simulink model "Third_Simulation"  (R2020a)
settings: Solver=VariableStepAuto  StartTime=0.0  StopTime=1  RelTol=1e-3
undefined symbols (not defined in the file): D1, Delta
libraries: powerlib x7
settings Model: Creator=amnja  LastModifiedBy=amnja

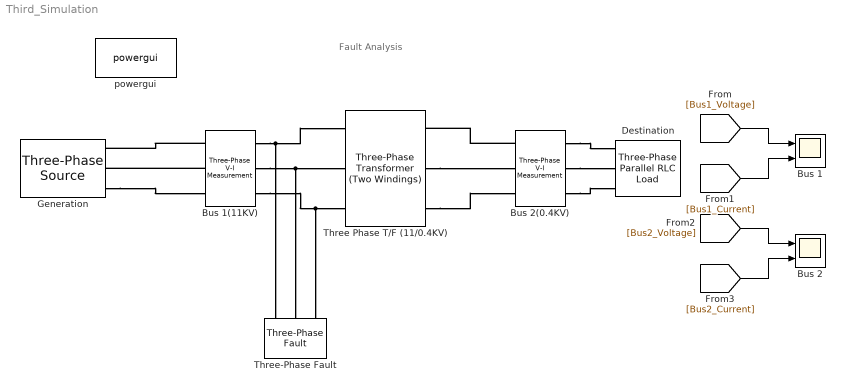
== system Third_Simulation ==
  note: Fault Analysis
  Bus 1 : Scope  NumInputPorts=2
  Bus 1(11KV) : powerlib/Measurements/Three-Phase V-I Measurement  VoltageMeasurement=phase-to-ground  SetLabelV=on  LabelV=Bus1_Voltage  Vpu=off  VpuLL=off  CurrentMeasurement=yes  SetLabelI=on  LabelI=Bus1_Current  Ipu=off  Pbase=100e6  Vbase=500e3  OutputType=Complex  PhasorSimulation=off  PSBequivalent=0
  Bus 2 : Scope  NumInputPorts=2
  Bus 2(0.4KV) : powerlib/Measurements/Three-Phase V-I Measurement  VoltageMeasurement=phase-to-ground  SetLabelV=on  LabelV=Bus2_Voltage  Vpu=off  VpuLL=off  CurrentMeasurement=yes  SetLabelI=on  LabelI=Bus2_Current  Ipu=off  Pbase=100e6  Vbase=500e3  OutputType=Complex  PhasorSimulation=off  PSBequivalent=0
  Destination : powerlib/Elements/Three-Phase Parallel RLC Load  LConnTagsString=A|B|C  Configuration=Y (grounded)  NominalVoltage=0.4e3  Vabc=[1e3 1e3 1e3]  Vabcp=[1e3 1e3 1e3]  NominalFrequency=50  UnbalancedPower=off  ActivePower=10e3  InductivePower=100  CapacitivePower=0  Pabc=[10e3 9e3 11e3]  QLabc=[100 90 110]  QCabc=[100 90 110]  Pabcp=[10e3 9e3 11e3]  QLabcp=[100 90 110]  QCabcp=[100 90 110]  Measurements=None  LoadType=constant Z
  Generation : powerlib/Electrical Sources/Three-Phase Source  InternalConnection=Yg  VoltagePhases=off  Voltage=11e3  PhaseAngle=0  Voltage_phases=[25e3 25e3 25e3]/sqrt(3)  PhaseAngles_phases=[0 -120 +120]  Frequency=50  NonIdealSource=on  SpecifyImpedance=off  Resistance=0.8929  Inductance=16.58e-3  ShortCircuitLevel=100e6  BaseVoltage=11e3  XRratio=7  BusType=PV  Pref=30e6  Qref=0  Prefabc=[10e3, 10e3, 10e3]  Qrefabc=[0, 0, 0]  Qmin=-inf  Qmax=inf
  Three Phase T/F (11/0.4KV) : powerlib/Elements/Three-Phase Transformer (Two Windings)  Winding1Connection=Delta (D1)  Winding2Connection=Yg  CoreType=Three single-phase transformers  SetSaturation=off  Hysteresis=off  DataFile='hysteresis'  SetInitialFlux=off  Measurements=None  UNITS=pu  NominalPower=[ 1e6 , 50 ]  Winding1=[ 11e3 , 0.002 , 0.08 ]  Winding2=[0.4e3 , 0.002 , 0.08 ]  Rm=500  Lm=500  L0=0.5  Saturation=[ 0,0 ; 0.0024,1.2 ; 1.0,1.52 ]  InitialFluxes=[ 0.8 , -0.8 , 0.7 ]  BreakLoop=off  DiscreteSolver=Trapezoidal iterative  DataType=off  TransfoNumber=1
  Three-Phase Fault : powerlib/Elements/Three-Phase Fault  InitialStates=0  FaultA=on  FaultB=off  FaultC=off  GroundFault=on  SwitchTimes="[1/50  5/50]"  External=off  SwitchStatus=NaN  FaultResistance=0.001  GroundResistance=0.01  SnubberResistance=1e6  SnubberCapacitance=inf  Measurements=None
  powergui : powerlib/powergui  Priority=1  SimulationMode=Continuous  SampleTime=50e-6  frequency=60  Iterations=50  frequencyindice=50  Pbase=100e6  ErrMax=1e-4  UnitsV=kV  UnitsW=MW  buscounter=0  FunctionMessages=off  echomessages=off  EnableUseOfTLC=off  CurrentSourceSwitches=off  DisableSnubberDevices=off  DisableRonSwitches=off  DisableVfSwitches=off  DisplayEquations=off  AutomaticDiscreteSolvers=off  SolverType=Tustin/Backward Euler (TBE)  Interpol=off  ExternalGateDelay=off  methode=off  Ts=100  x0status=blocks  SPID=on  SwTol=0  HookPort=off  NonlinearTolerance=1e-4  nMaxIteration=100  ContinueOnMaxIteration=off  RestoreLinks=warning  ResistiveCurrentMeasurement=off  Frange=[0:2:500]  Ylog=off  Xlog=on  ShowGrid=off  save=off  variable=ZData  structure=0  ZoomFFT=off  StartTime=0.0  cycles=1  DisplayStyle=1  fundamental=60  FreqAxis=off  MaxFrequency=1000  frequencyindicesteady=1  RmsSteady=1  display=off
  wires:
  [Bus1_Voltage] -> Bus 1/1
  [Bus1_Current] -> Bus 1/2
  [Bus2_Current] -> Bus 2/2
  [Bus2_Voltage] -> Bus 2/1
  connections:
  Bus 1(11KV)/RConn1 -- Three Phase T/F (11/0.4KV)/LConn1 -- Three-Phase Fault/LConn1
  Bus 1(11KV)/LConn2 -- Generation/RConn2
  Bus 1(11KV)/LConn1 -- Generation/RConn1
  Generation/RConn3 -- Bus 1(11KV)/LConn3
  Bus 1(11KV)/RConn2 -- Three Phase T/F (11/0.4KV)/LConn2 -- Three-Phase Fault/LConn2
  Bus 1(11KV)/RConn3 -- Three Phase T/F (11/0.4KV)/LConn3 -- Three-Phase Fault/LConn3
  Bus 2(0.4KV)/LConn1 -- Three Phase T/F (11/0.4KV)/RConn1
  Three Phase T/F (11/0.4KV)/RConn2 -- Bus 2(0.4KV)/LConn2
  Three Phase T/F (11/0.4KV)/RConn3 -- Bus 2(0.4KV)/LConn3
  Bus 2(0.4KV)/RConn1 -- Destination/LConn1
  Bus 2(0.4KV)/RConn2 -- Destination/LConn2
  Bus 2(0.4KV)/RConn3 -- Destination/LConn3
